simulink model "Versal_RF_Channelizer_Ex1"  (R2025a)
settings: Solver=VariableStepAuto  StopTime=4000/100e6
InitFcn:
  | num_chan = 8;  % Number of channels
  | taps_per_phase = 20; % Number of taps per channel.
  | count = 1;
  | for i=0:1:num_chan-1 % number of channels
  |       coeffs_set_num(count:count+taps_per_phase+2) = i;
  |       count = count + taps_per_phase+2;
  |      if i == 0
  |        coeffs_set_num(count:count+5) = 0;
  |        count = count + 5;
  |      else
  |        coeffs_set_num(count:count+2) = 0;
  |        count = count + 2;
  |     end
  | 
  | end
  | 
  | coeffs_set_num = coeffs_set_num(1:160);
  | coeffs_tlast = [zeros(1,num_chan)];
  | for k=1:1:39
  | coeffs_tlast = [coeffs_tlast,1,zeros(1,(num_chan/2)-1)];
  | end
  | coeffs_tlast = coeffs_tlast(1:160);
undefined symbols (not defined in the file): S, vsva2488, xcvr1602
libraries: hdlBasic x27, dspsrcs4 x4, dspswit3 x2, hdlDSPIP x1, vmcUtilities x1
settings Model: Creator=nanumolu  LastModifiedBy=robg

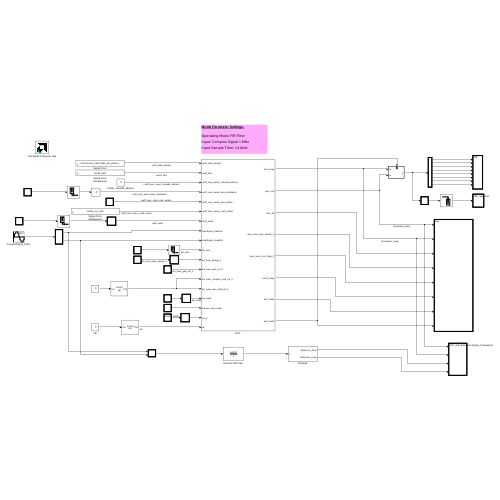
[thumbnail: Simulink's stored preview of the top-level diagram]
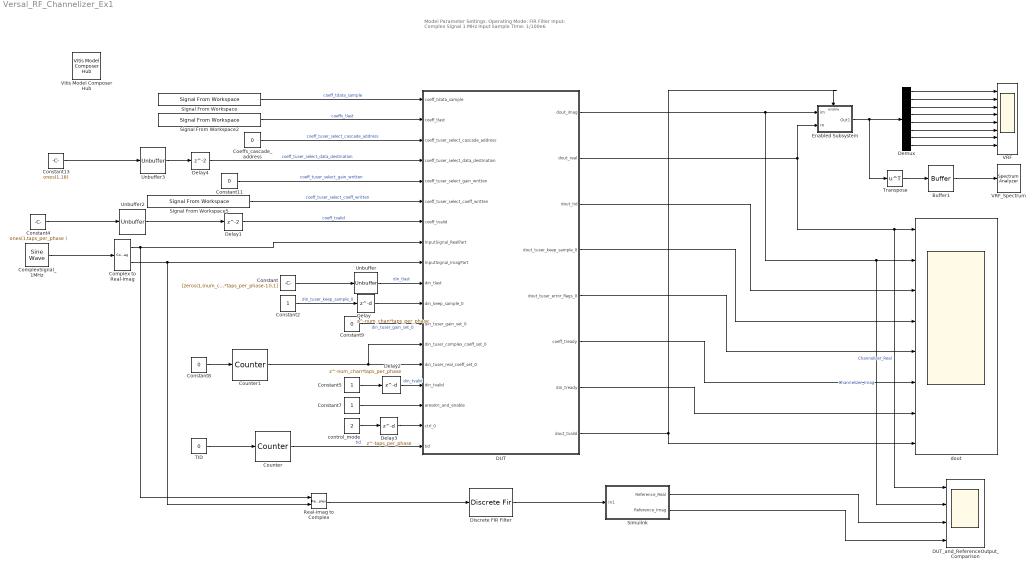
== system Versal_RF_Channelizer_Ex1 ==
  note: Model Parameter Settings:
      |
      | Operating Mode: FIR Filter
      | Input: Complex Signal 1 MHz
      | Input Sample TIme: 1/100e6
  Buffer1 : Buffer  N=1024  OutputFrames=off
  Coeffs_cascade_address : Constant  Value=0  SampleTime=1/100e6
  Complex to Real-Imag : ComplexToRealImag
  ComplexSignal_1MHz : dspsrcs4/Sine Wave  Amplitude=0.15  Frequency=1e6  Phase=0  SampleMode=Discrete  OutComplex=Complex  CompMethod=Trigonometric fcn  TableSize=Speed  SampleTime=1/100e6  SamplesPerFrame=1  ResetState=Restart at time zero  OutputFrames=off  dataType=double  wordLen=16  udDataType=sfix(16)  fracBitsMode=Best precision  numFracBits=15  OutDataTypeStr=double  LastOutDataTypeStr=double
  Constant : Constant  Value=[zeros(1,(num_chan*taps_per_phase-1)),1]  SampleTime=1/100e6
  Constant11 : Constant  Value=0  SampleTime=1/100e6
  Constant13 : Constant  Value=ones(1,18)  SampleTime=1/100e6
  Constant2 : Constant  SampleTime=1/100e6
  Constant4 : Constant  Value=ones(1,taps_per_phase )  SampleTime=1/100e6
  Constant5 : Constant  SampleTime=1/100e6
  Constant7 : Constant  SampleTime=1/100e6
  Constant8 : Constant  Value=0  SampleTime=1/100e6
  Constant9 : Constant  Value=0  SampleTime=1/100e6
  Counter : dspswit3/Counter  Direction=Up  CountEvent=Rising edge  CounterSize=User defined  MaxCount=num_chan-1  InitialCount=0  Output=Count  HitValue=32  ResetInput=off  SamplesPerFrame=1  Ts=1  CntDtype=double  HitDtype=Logical
  Counter1 : dspswit3/Counter  Direction=Up  CountEvent=Rising edge  CounterSize=User defined  MaxCount=num_chan-1  InitialCount=0  Output=Count  HitValue=32  ResetInput=off  SamplesPerFrame=1  Ts=1  CntDtype=double  HitDtype=Logical
  DUT : Subsystem
  DUT_and_ReferenceOutput_Comparison : Scope  NumInputPorts=4
      settings: ActiveDisplayYMinimum=-0.4404  ActiveDisplayYMaximum=0.4404
  Delay : Delay  DelayLength=num_chan*taps_per_phase
  Delay1 : Delay
  Delay2 : Delay  DelayLength=num_chan*taps_per_phase
  Delay3 : Delay  DelayLength=taps_per_phase
  Delay4 : Delay
  Demux : Demux  Outputs=8
  Discrete FIR Filter : DiscreteFir  Coefficients=ones(1,20)  InputProcessing=Columns as channels (frame based)  OutDataTypeStr=Inherit: Same as input
  Enabled Subsystem : Subsystem  TreatAsAtomicUnit=on
  Real-Imag to Complex : RealImagToComplex
  Signal From Workspace : dspsrcs4/Signal From Workspace  X=ones(1,num_chan*taps_per_phase )  Ts=1/100e6  nsamps=1  OutputAfterFinalValue=Setting to zero  ignoreOrWarnInputAndFrameLengths=off  OutputFrames=off
  Signal From Workspace2 : dspsrcs4/Signal From Workspace  X=coeffs_tlast  Ts=1/100e6  nsamps=1  OutputAfterFinalValue=Setting to zero  ignoreOrWarnInputAndFrameLengths=off  OutputFrames=off
  Signal From Workspace5 : dspsrcs4/Signal From Workspace  X=coeffs_set_num  Ts=1/100e6  nsamps=1  OutputAfterFinalValue=Setting to zero  ignoreOrWarnInputAndFrameLengths=off  OutputFrames=off
  Simulink : Subsystem
  TID : Constant  Value=0  SampleTime=1
  Transpose : Math  Operator=transpose
  Unbuffer : Unbuffer
  Unbuffer2 : Unbuffer
  Unbuffer3 : Unbuffer
  VRF : Scope  NumInputPorts=8
      settings: TimeUnits=Metric (based on Time Span)  ActiveDisplayYMinimum=-0.4404  ActiveDisplayYMaximum=0.4404  YLabel=Amplitude  DataLoggingVariableName=ScopeData3
  VRF_Spectrum : SpectrumAnalyzer  WindowPosition=[1.000000,1.000000,1920.000000,1127.000000,]  ScopeFrameLocation=window  Span=100000000  StartFrequency=-50000000  StopFrequency=50000000  YLimits=[-87.1326 27.2272]
  Vitis Model Composer Hub : vmcUtilities/Vitis Model Composer Hub  Tag=genX  CodeGeneration=off  SubsystemName=DUT  BlockHierPath=Channalizer_smoke  CompilationType=HDLCompilation  SubsystemType=HDLNode  ExportTypeV2=HDL Netlist  StartColumn=1  NumberOfColumns=1  TargetDirectory=./netlist_chan_vlg  exportDesign=on  analyzeDesign=off  validateDesignOnHw=off  ExportType=AI Engines  IpVendor=xilinx.com  IpLibrary=hls  IpVersion=1.0  IpHWLanguage=Verilog  AieCompilerOptions={}  AieSimulatorOptions={}  CreateTestbench=on  TestbenchStackSize=10  RunRtlSim=off  RunCSim=off  RunAieSim=off  enableSimulationTimeout=on  enableGraphIterations=on  AieSimTimeout=50000  AieGraphIterations=-1  RunAieSimProfiling=off  LaunchVitisAnalyzer=off  PlotOutput=off  RunX86Sim=off  X86SimTimeout=10  GenHwImage=off  GenLibadfXo=on  GenHwValidationCode=off  PlatformType=Not Specified  HwSystemType=Baremetal  HwValidationTarget=hw  ProjDevice=xcvr1602-vsva2488-2MP-e-S  ProjDevicePart=xcvr1602-vsva2488-2MP-e-S  AIEType=AIE  SamplePeriod=-1  ClockFrequency=200  DataPathParallelism=1  xilinxfamily=versalrf  part=xcvr1602  speed=-2MP-e-S  package=vsva2488  directory=./netlist/ip/DUT/src  testbench=off  incr_netlist=off  synthesis_tool=Vivado  clock_wrapper=Clock Enables  dbl_ovrd=According to Block Masks  dcm_input_clock_period=10  sysclk_period=10  simulink_period=1/100e6  eval_field=0  IPInfoJsonString="{\"DUTSubsystemName\":\"Channalizer_smoke\",\"HDLSubsystem\":{\"SubsystemName\":\"Channalizer_smoke\",\"IPName\":\"Copy_of_hamilton_vrf_fft\",\"IPLibrary\":\"VMC\",\"IPVendor\":\"User Company\",\"IPVersion\":\"1.0\",\"TargetDirectory\":\"./netlist_chan_vlg\",\"SubsystemDir\":\"./netlist_chan_vlg/ip/Channalizer_smoke\",\"FreqHz\":\"100000000\"},\"SubsystemTag\":\"HDLNode\"}"  LogFileName=/proj/dsv_xhd/ravalib/Head/Tests/REL/2025.1/dsv/modelcomposer/hdl/regression/channelizer/smoke/netlist_chan_vlg/model_composer.log  NThreads=4  IPConfigFile=/tmp/vmctmp-10364637636032824832/Channalizer_smoke_ipconfig.json
  control_mode : Constant  Value=2  SampleTime=1/100e6
  dout : Scope  NumInputPorts=8
      settings: ActiveDisplayYMinimum=-0.4404  ActiveDisplayYMaximum=0.4404
  wires:
  Signal From Workspace/1 -> DUT/1(coeff_tdata_sample)  "coeff_tdata_sample"
  Constant11/1 -> DUT/5(coeff_tuser_select_gain_written)  "coeff_tuser_select_gain_written"
  Coeffs_cascade_address/1 -> DUT/3(coeff_tuser_select_cascade_address)  "coeff_tuser_select_cascade_address"
  Delay4/1 -> DUT/4(coeff_tuser_select_data_destination)  "coeff_tuser_select_data_destination"
  Delay1/1 -> DUT/7(coeff_tvalid)  "coeff_tvalid"
  Unbuffer/1 -> DUT/10(din_tlast)  "din_tlast"
  Constant2/1 -> Delay/1  "din_tuser_keep_sample_0"
  Counter1/1 -> DUT/13(din_tuser_complex_coeff_set_0), DUT/14(din_tuser_real_coeff_set_0)
  Complex to Real-Imag/2 -> DUT/9(InputSignal_ImagPart), Real-Imag to Complex/2
  Constant/1 -> Unbuffer/1
  TID/1 -> Counter/1
  Constant4/1 -> Unbuffer2/1
  Unbuffer2/1 -> Delay1/1
  Constant5/1 -> Delay2/1
  control_mode/1 -> Delay3/1
  Constant8/1 -> Counter1/1
  Constant13/1 -> Unbuffer3/1
  Unbuffer3/1 -> Delay4/1
  DUT/2(dout_real) -> DUT_and_ReferenceOutput_Comparison/1, dout/1, Enabled Subsystem/2(re)  "Channelizer_Real"
  DUT/1(dout_imag) -> Enabled Subsystem/1(im), dout/2, DUT_and_ReferenceOutput_Comparison/2  "Channelizer_Imag"
  Signal From Workspace5/1 -> DUT/6(coeff_tuser_select_coeff_written)  "coeff_tuser_select_coeff_written"
  DUT/3(dout_tid) -> dout/3
  DUT/4(dout_tuser_keep_sample_0) -> dout/4
  DUT/5(dout_tuser_error_flags_0) -> dout/5
  DUT/6(coeff_tready) -> dout/6
  DUT/7(din_tready) -> dout/7
  Enabled Subsystem/1(Out1) -> Demux/1, Transpose/1
  Buffer1/1 -> VRF_Spectrum/1
  Signal From Workspace2/1 -> DUT/2(coeff_tlast)  "coeffs_tlast"
  Transpose/1 -> Buffer1/1
  Demux/1 -> VRF/1
  Demux/2 -> VRF/2
  Demux/3 -> VRF/3
  Demux/4 -> VRF/4
  Demux/5 -> VRF/5
  Demux/6 -> VRF/6
  Demux/7 -> VRF/7
  Demux/8 -> VRF/8
  Real-Imag to Complex/1 -> Discrete FIR Filter/1
  Delay3/1 -> DUT/17(ctrl_0)
  Counter/1 -> DUT/18(tid)  "tid"
  Complex to Real-Imag/1 -> DUT/8(InputSignal_RealPart), Real-Imag to Complex/1
  Delay2/1 -> DUT/15(din_tvalid)  "din_tvalid"
  Constant7/1 -> DUT/16(aresetn_and_enable)
  Constant9/1 -> DUT/12(din_tuser_gain_set_0)  "din_tuser_gain_set_0"
  Delay/1 -> DUT/11(din_keep_sample_0)
  DUT/8(dout_tvalid) -> dout/8, Enabled Subsystem/Enable
  Discrete FIR Filter/1 -> Simulink/1(In1)
  Simulink/1(Reference_Real) -> DUT_and_ReferenceOutput_Comparison/3
  Simulink/2(Reference_Imag) -> DUT_and_ReferenceOutput_Comparison/4
  ComplexSignal_1MHz/1 -> Complex to Real-Imag/1

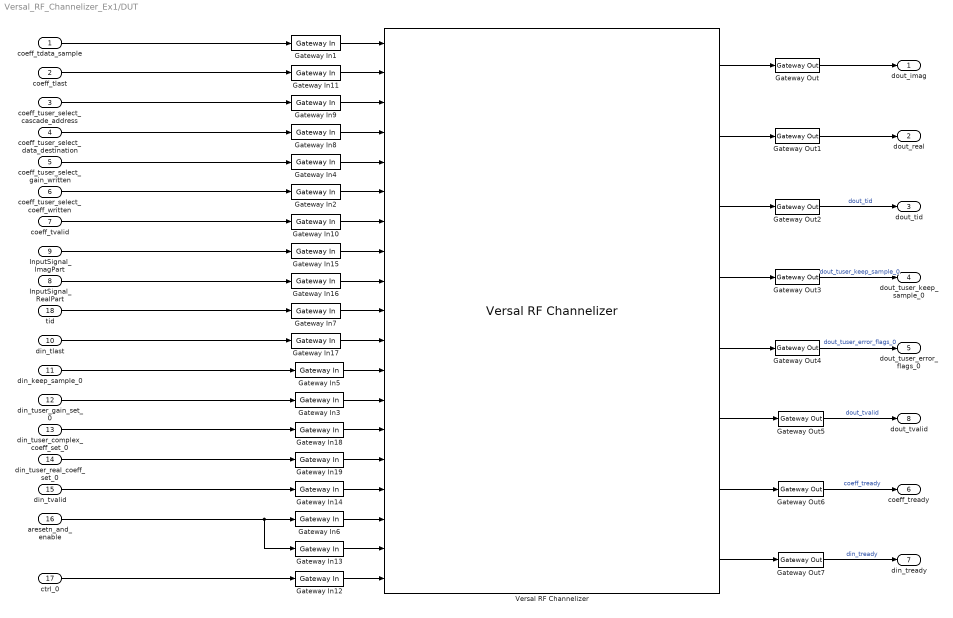
== system Versal_RF_Channelizer_Ex1/DUT ==
  coeff_tdata_sample : Inport
  coeff_tlast : Inport  Port=2
  coeff_tuser_select_cascade_address : Inport  Port=3
  coeff_tuser_select_data_destination : Inport  Port=4
  coeff_tuser_select_gain_written : Inport  Port=5
  coeff_tuser_select_coeff_written : Inport  Port=6
  coeff_tvalid : Inport  Port=7
  InputSignal_RealPart : Inport  Port=8
  InputSignal_ImagPart : Inport  Port=9
  din_tlast : Inport  Port=10
  din_keep_sample_0 : Inport  Port=11
  din_tuser_gain_set_0 : Inport  Port=12
  din_tuser_complex_coeff_set_0 : Inport  Port=13
  din_tuser_real_coeff_set_0 : Inport  Port=14
  din_tvalid : Inport  Port=15
  aresetn_and_enable : Inport  Port=16
  ctrl_0 : Inport  Port=17
  tid : Inport  Port=18
  Gateway In1 : hdlBasic/Gateway In  gui_display_data_type=Fixed-point  arith_type=Signed (2's comp)  n_bits=18  bin_pt=17  preci_type=Single  exp_width=8  frac_width=24  rows=1  columns=1  quantization="Round  (unbiased: +/- Inf)"  overflow=Saturate  period=1/100e6  UseAsADC=off  ADCChannel='1'  interface=None  automatic_assignment=on  address_offset=hex2dec('00')  intf_name=''  intf_description=''  default_value=0  timing_constraint=None  locs_specified=off  LOCs={}  io_standard={}  inherit_from_input=off  hdl_port=on  XmcBlockStatus=1  maskContainerNames=group4  block_type=gatewayin  block_config=sysgen:gateway_in_config  block_width_w=590  block_height_w=620  block_width=640  block_height=850
  Gateway In{6,10..11,13..14,17} (6 alike) : hdlBasic/Gateway In  gui_display_data_type=Boolean  arith_type=Boolean  n_bits=16  bin_pt=14  preci_type=Single  exp_width=8  frac_width=24  rows=1  columns=1  quantization="Round  (unbiased: +/- Inf)"  overflow=Saturate  period=1/100e6  UseAsADC=off  ADCChannel='1'  interface=None  automatic_assignment=on  address_offset=hex2dec('00')  intf_name=''  intf_description=''  default_value=0  timing_constraint=None  locs_specified=off  LOCs={}  io_standard={}  inherit_from_input=off  hdl_port=on  XmcBlockStatus=1  maskContainerNames=group4  block_type=gatewayin  block_config=sysgen:gateway_in_config  block_width_w=590  block_height_w=620  block_width=640  block_height=850
  Gateway In12 : hdlBasic/Gateway In  gui_display_data_type=Fixed-point  arith_type=Signed (2's comp)  n_bits=8  bin_pt=0  preci_type=Single  exp_width=8  frac_width=24  rows=1  columns=1  quantization="Round  (unbiased: +/- Inf)"  overflow=Saturate  period=1/100e6  UseAsADC=off  ADCChannel='1'  interface=None  automatic_assignment=on  address_offset=hex2dec('00')  intf_name=''  intf_description=''  default_value=0  timing_constraint=None  locs_specified=off  LOCs={}  io_standard={}  inherit_from_input=off  hdl_port=on  XmcBlockStatus=1  maskContainerNames=group4  block_type=gatewayin  block_config=sysgen:gateway_in_config  block_width_w=590  block_height_w=620  block_width=640  block_height=850
  Gateway In15 : hdlBasic/Gateway In  gui_display_data_type=Fixed-point  arith_type=Signed (2's comp)  n_bits=18  bin_pt=17  preci_type=Single  exp_width=8  frac_width=24  rows=1  columns=1  quantization="Round  (unbiased: +/- Inf)"  overflow=Saturate  period=1/100e6  UseAsADC=off  ADCChannel='1'  interface=None  automatic_assignment=on  address_offset=hex2dec('00')  intf_name=''  intf_description=''  default_value=0  timing_constraint=None  locs_specified=off  LOCs={}  io_standard={}  inherit_from_input=off  hdl_port=on  XmcBlockStatus=1  maskContainerNames=group4  block_type=gatewayin  block_config=sysgen:gateway_in_config  block_width_w=590  block_height_w=620  block_width=640  block_height=850
  Gateway In16 : hdlBasic/Gateway In  gui_display_data_type=Fixed-point  arith_type=Signed (2's comp)  n_bits=18  bin_pt=17  preci_type=Single  exp_width=8  frac_width=24  rows=1  columns=1  quantization="Round  (unbiased: +/- Inf)"  overflow=Saturate  period=1/100e6  UseAsADC=off  ADCChannel='1'  interface=None  automatic_assignment=on  address_offset=hex2dec('00')  intf_name=''  intf_description=''  default_value=0  timing_constraint=None  locs_specified=off  LOCs={}  io_standard={}  inherit_from_input=off  hdl_port=on  XmcBlockStatus=1  maskContainerNames=group4  block_type=gatewayin  block_config=sysgen:gateway_in_config  block_width_w=590  block_height_w=620  block_width=640  block_height=850
  Gateway In18 : hdlBasic/Gateway In  gui_display_data_type=Fixed-point  arith_type=Unsigned  n_bits=3  bin_pt=0  preci_type=Single  exp_width=8  frac_width=24  rows=1  columns=1  quantization="Round  (unbiased: +/- Inf)"  overflow=Saturate  period=1/100e6  UseAsADC=off  ADCChannel='1'  interface=None  automatic_assignment=on  address_offset=hex2dec('00')  intf_name=''  intf_description=''  default_value=0  timing_constraint=None  locs_specified=off  LOCs={}  io_standard={}  inherit_from_input=off  hdl_port=on  XmcBlockStatus=1  maskContainerNames=group4  block_type=gatewayin  block_config=sysgen:gateway_in_config  block_width_w=590  block_height_w=620  block_width=640  block_height=850
  Gateway In19 : hdlBasic/Gateway In  gui_display_data_type=Fixed-point  arith_type=Unsigned  n_bits=3  bin_pt=0  preci_type=Single  exp_width=8  frac_width=24  rows=1  columns=1  quantization="Round  (unbiased: +/- Inf)"  overflow=Saturate  period=1/100e6  UseAsADC=off  ADCChannel='1'  interface=None  automatic_assignment=on  address_offset=hex2dec('00')  intf_name=''  intf_description=''  default_value=0  timing_constraint=None  locs_specified=off  LOCs={}  io_standard={}  inherit_from_input=off  hdl_port=on  XmcBlockStatus=1  maskContainerNames=group4  block_type=gatewayin  block_config=sysgen:gateway_in_config  block_width_w=590  block_height_w=620  block_width=640  block_height=850
  Gateway In2 : hdlBasic/Gateway In  gui_display_data_type=Fixed-point  arith_type=Unsigned  n_bits=3  bin_pt=0  preci_type=Single  exp_width=8  frac_width=24  rows=1  columns=1  quantization="Round  (unbiased: +/- Inf)"  overflow=Saturate  period=1/100e6  UseAsADC=off  ADCChannel='1'  interface=None  automatic_assignment=on  address_offset=hex2dec('00')  intf_name=''  intf_description=''  default_value=0  timing_constraint=None  locs_specified=off  LOCs={}  io_standard={}  inherit_from_input=off  hdl_port=on  XmcBlockStatus=1  maskContainerNames=group4  block_type=gatewayin  block_config=sysgen:gateway_in_config  block_width_w=590  block_height_w=620  block_width=640  block_height=850
  Gateway In3 : hdlBasic/Gateway In  gui_display_data_type=Fixed-point  arith_type=Unsigned  n_bits=1  bin_pt=0  preci_type=Single  exp_width=8  frac_width=24  rows=1  columns=1  quantization="Round  (unbiased: +/- Inf)"  overflow=Saturate  period=1/100e6  UseAsADC=off  ADCChannel='1'  interface=None  automatic_assignment=on  address_offset=hex2dec('00')  intf_name=''  intf_description=''  default_value=0  timing_constraint=None  locs_specified=off  LOCs={}  io_standard={}  inherit_from_input=off  hdl_port=on  XmcBlockStatus=1  maskContainerNames=group4  block_type=gatewayin  block_config=sysgen:gateway_in_config  block_width_w=590  block_height_w=620  block_width=640  block_height=850
  Gateway In4 : hdlBasic/Gateway In  gui_display_data_type=Fixed-point  arith_type=Unsigned  n_bits=1  bin_pt=0  preci_type=Single  exp_width=8  frac_width=24  rows=1  columns=1  quantization="Round  (unbiased: +/- Inf)"  overflow=Saturate  period=1/100e6  UseAsADC=off  ADCChannel='1'  interface=None  automatic_assignment=on  address_offset=hex2dec('00')  intf_name=''  intf_description=''  default_value=0  timing_constraint=None  locs_specified=off  LOCs={}  io_standard={}  inherit_from_input=off  hdl_port=on  XmcBlockStatus=1  maskContainerNames=group4  block_type=gatewayin  block_config=sysgen:gateway_in_config  block_width_w=590  block_height_w=620  block_width=640  block_height=850
  Gateway In5 : hdlBasic/Gateway In  gui_display_data_type=Fixed-point  arith_type=Unsigned  n_bits=1  bin_pt=0  preci_type=Single  exp_width=8  frac_width=24  rows=1  columns=1  quantization="Round  (unbiased: +/- Inf)"  overflow=Saturate  period=1/100e6  UseAsADC=off  ADCChannel='1'  interface=None  automatic_assignment=on  address_offset=hex2dec('00')  intf_name=''  intf_description=''  default_value=0  timing_constraint=None  locs_specified=off  LOCs={}  io_standard={}  inherit_from_input=off  hdl_port=on  XmcBlockStatus=1  maskContainerNames=group4  block_type=gatewayin  block_config=sysgen:gateway_in_config  block_width_w=590  block_height_w=620  block_width=640  block_height=850
  Gateway In7 : hdlBasic/Gateway In  gui_display_data_type=Fixed-point  arith_type=Signed (2's comp)  n_bits=3  bin_pt=0  preci_type=Single  exp_width=8  frac_width=24  rows=1  columns=1  quantization="Round  (unbiased: +/- Inf)"  overflow=Saturate  period=1/100e6  UseAsADC=off  ADCChannel='1'  interface=None  automatic_assignment=on  address_offset=hex2dec('00')  intf_name=''  intf_description=''  default_value=0  timing_constraint=None  locs_specified=off  LOCs={}  io_standard={}  inherit_from_input=off  hdl_port=on  XmcBlockStatus=1  maskContainerNames=group4  block_type=gatewayin  block_config=sysgen:gateway_in_config  block_width_w=590  block_height_w=620  block_width=640  block_height=850
  Gateway In8 : hdlBasic/Gateway In  gui_display_data_type=Fixed-point  arith_type=Unsigned  n_bits=2  bin_pt=0  preci_type=Single  exp_width=8  frac_width=24  rows=1  columns=1  quantization="Round  (unbiased: +/- Inf)"  overflow=Saturate  period=1/100e6  UseAsADC=off  ADCChannel='1'  interface=None  automatic_assignment=on  address_offset=hex2dec('00')  intf_name=''  intf_description=''  default_value=0  timing_constraint=None  locs_specified=off  LOCs={}  io_standard={}  inherit_from_input=off  hdl_port=on  XmcBlockStatus=1  maskContainerNames=group4  block_type=gatewayin  block_config=sysgen:gateway_in_config  block_width_w=590  block_height_w=620  block_width=640  block_height=850
  Gateway In9 : hdlBasic/Gateway In  gui_display_data_type=Fixed-point  arith_type=Unsigned  n_bits=4  bin_pt=0  preci_type=Single  exp_width=8  frac_width=24  rows=1  columns=1  quantization="Round  (unbiased: +/- Inf)"  overflow=Saturate  period=1/100e6  UseAsADC=off  ADCChannel='1'  interface=None  automatic_assignment=on  address_offset=hex2dec('00')  intf_name=''  intf_description=''  default_value=0  timing_constraint=None  locs_specified=off  LOCs={}  io_standard={}  inherit_from_input=off  hdl_port=on  XmcBlockStatus=1  maskContainerNames=group4  block_type=gatewayin  block_config=sysgen:gateway_in_config  block_width_w=590  block_height_w=620  block_width=640  block_height=850
  Gateway Out{,1..7} (8 alike) : hdlBasic/Gateway Out  inherit_from_input=off  bool_to_boolean=off  hdl_port=on  rows=1  columns=1  UseAsDAC=off  DACChannel='1'  interface=None  automatic_assignment=on  address_offset=hex2dec('00')  intf_name=''  intf_description=''  timing_constraint=None  locs_specified=off  LOCs={}  io_standard={}  XmcBlockStatus=1  maskContainerNames=group4  block_type=gatewayout  block_config=sysgen:gateway_out_config  block_width_w=590  block_height_w=620  block_width=620  block_height=750
  Versal RF Channelizer : hdlDSPIP/Versal RF Channelizer  mode=FIR Filter  input_sample_rate=1  num_of_instances=1  fft_direction=FFT  fft_sync_on_tlast=off  fir_coeff_type=Real  fir_length=16  gain_en=off  events=off  coeff_casc_en=off  active_duty_cycle=25  toggle_rate=25  fir_unit_0_taps=16  fir_unit_1_taps=0  fir_unit_2_taps=0  fir_unit_3_taps=0  ip_name=Versal RF Channelizer  enable_all_ports=false  ip_version=1.2  dsptool_ready=false  ipcore_usecache=true  ipcore_useipmodelcache=true  wrapper_available=true  port_translation_map={ 'aclken' => 'en', 'aresetn' => 'rst' }  structural_sim=true  ipcore_do_not_force_period=true  oldconvolution_code_radix=Binary  XmcBlockStatus=1  maskContainerNames=tabcontainer1  block_type=vrf_channelizer_v1_1  block_config=sysgen:rodinimport_config
  dout_imag : Outport
  dout_real : Outport  Port=2
  dout_tid : Outport  Port=3
  dout_tuser_keep_sample_0 : Outport  Port=4
  dout_tuser_error_flags_0 : Outport  Port=5
  coeff_tready : Outport  Port=6
  din_tready : Outport  Port=7
  dout_tvalid : Outport  Port=8
  wires:
  Gateway In11/1 -> Versal RF Channelizer/2
  Gateway In8/1 -> Versal RF Channelizer/4
  coeff_tuser_select_coeff_written/1 -> Gateway In2/1
  Gateway In9/1 -> Versal RF Channelizer/3
  Gateway In15/1 -> Versal RF Channelizer/8
  Versal RF Channelizer/4 -> Gateway Out3/1
  Versal RF Channelizer/6 -> Gateway Out5/1
  din_tuser_complex_coeff_set_0/1 -> Gateway In18/1
  Versal RF Channelizer/1 -> Gateway Out/1
  Gateway In13/1 -> Versal RF Channelizer/18
  Versal RF Channelizer/8 -> Gateway Out7/1
  Gateway Out2/1 -> dout_tid/1  "dout_tid"
  coeff_tuser_select_gain_written/1 -> Gateway In4/1
  Gateway In19/1 -> Versal RF Channelizer/15
  Gateway In1/1 -> Versal RF Channelizer/1
  Versal RF Channelizer/7 -> Gateway Out6/1
  Gateway Out1/1 -> dout_real/1
  InputSignal_ImagPart/1 -> Gateway In15/1
  Gateway In12/1 -> Versal RF Channelizer/19
  din_tuser_gain_set_0/1 -> Gateway In3/1
  coeff_tlast/1 -> Gateway In11/1
  Gateway In6/1 -> Versal RF Channelizer/17
  ctrl_0/1 -> Gateway In12/1
  Gateway In18/1 -> Versal RF Channelizer/14
  din_tuser_real_coeff_set_0/1 -> Gateway In19/1
  InputSignal_RealPart/1 -> Gateway In16/1
  din_tvalid/1 -> Gateway In14/1
  coeff_tuser_select_data_destination/1 -> Gateway In8/1
  Gateway In2/1 -> Versal RF Channelizer/6
  Versal RF Channelizer/3 -> Gateway Out2/1
  coeff_tuser_select_cascade_address/1 -> Gateway In9/1
  Versal RF Channelizer/2 -> Gateway Out1/1
  coeff_tvalid/1 -> Gateway In10/1
  Gateway In5/1 -> Versal RF Channelizer/12
  coeff_tdata_sample/1 -> Gateway In1/1
  Gateway In14/1 -> Versal RF Channelizer/16
  Gateway Out7/1 -> din_tready/1  "din_tready"
  Gateway In3/1 -> Versal RF Channelizer/13
  din_tlast/1 -> Gateway In17/1
  Gateway Out5/1 -> dout_tvalid/1  "dout_tvalid"
  din_keep_sample_0/1 -> Gateway In5/1
  Gateway Out/1 -> dout_imag/1
  Versal RF Channelizer/5 -> Gateway Out4/1
  Gateway In16/1 -> Versal RF Channelizer/9
  aresetn_and_enable/1 -> Gateway In13/1, Gateway In6/1
  Gateway In17/1 -> Versal RF Channelizer/11
  Gateway Out3/1 -> dout_tuser_keep_sample_0/1  "dout_tuser_keep_sample_0"
  Gateway Out6/1 -> coeff_tready/1  "coeff_tready"
  Gateway Out4/1 -> dout_tuser_error_flags_0/1  "dout_tuser_error_flags_0"
  Gateway In10/1 -> Versal RF Channelizer/7
  Gateway In4/1 -> Versal RF Channelizer/5
  tid/1 -> Gateway In7/1
  Gateway In7/1 -> Versal RF Channelizer/10

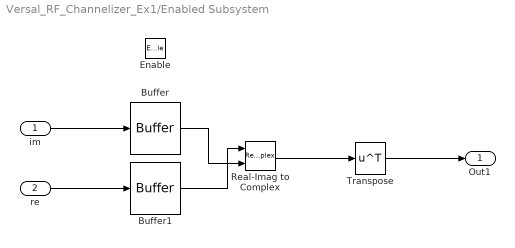
== system Versal_RF_Channelizer_Ex1/Enabled Subsystem ==
  im : Inport
  re : Inport  Port=2
  Enable : EnablePort
  Buffer : Buffer  N=num_chan  OutputFrames=off
  Buffer1 : Buffer  N=num_chan  OutputFrames=off
  Real-Imag to Complex : RealImagToComplex
  Transpose : Math  Operator=transpose
  Out1 : Outport
  wires:
  re/1 -> Buffer1/1
  im/1 -> Buffer/1
  Buffer/1 -> Real-Imag to Complex/2
  Buffer1/1 -> Real-Imag to Complex/1
  Real-Imag to Complex/1 -> Transpose/1
  Transpose/1 -> Out1/1

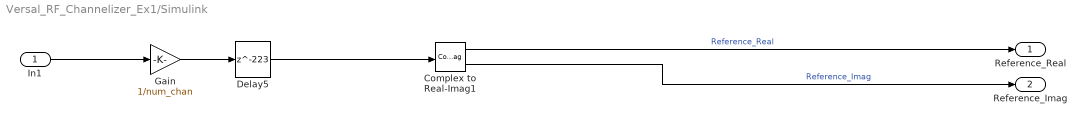
== system Versal_RF_Channelizer_Ex1/Simulink ==
  In1 : Inport
  Complex to Real-Imag1 : ComplexToRealImag
  Delay5 : Delay  DelayLength=223  DelayLengthUpperLimit=1000
  Gain : Gain  Gain=1/num_chan
  Reference_Real : Outport
  Reference_Imag : Outport  Port=2
  wires:
  Gain/1 -> Delay5/1
  Delay5/1 -> Complex to Real-Imag1/1
  Complex to Real-Imag1/1 -> Reference_Real/1  "Reference_Real"
  Complex to Real-Imag1/2 -> Reference_Imag/1  "Reference_Imag"
  In1/1 -> Gain/1
